simulink model "TDEKF"  (R2020a)
settings: Solver=FixedStepAuto  StartTime=0.0  StopTime=t_sim  FixedStep=0.001  RelTol=1e-3
undefined symbols (not defined in the file or in its folder): initial_acc, initial_position, initial_velocity
libraries: simulink x2
settings Model: Creator=addsd  LastModifiedBy=addsd
settings SFSimCC: CustomCodeUndefinedFunction=UseInterfaceOnly

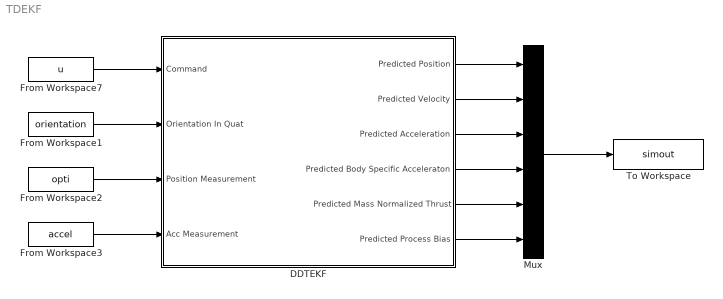
== system TDEKF ==
  DDTEKF : Subsystem  TreatAsAtomicUnit=on  mask{pos_init=initial_position, vel_init=initial_velocity, bsa_init=initial_acc, P_init=eye(11)*0.1, sig_acc=[0.0106 0.0116 0.02554], sig_pos=[0.00001 0.00001 0.00001], sig_quat=[0.001 0.001 0.001 0.001], sig_u=0.001}
      mask prompts: pos_init "Initial Position"; vel_init "Initial Velocity"; bsa_init "Initial Body Specific Acceleration"; P_init "Initial Covariance"; sig_acc "Accelerometer Variance"; sig_pos "Position Sensor Variance"; sig_quat "Orientation Measurement Variance"; sig_u "Process Variance"
      mask help:
      | DDTEKF For Qdrone 1234, dt set to 0.001, gravity vector set to [0 0 9.78909]
      | The Identified Parameters:
      | Kmz = 0.294861
      | Tmz = 0.017707
      | Td = [1.1629 1.1629 0.579374]
      mask init:
      | x_init = [pos_init vel_init bsa_init 5.8033 0]';
      | Q = diag([sig_u sig_quat]);
      | Q_tune = eye(11)*1e-6;
      | Q_tune(1:3, 1:3) = eye(3)*1e-6;
      | Q_tune(4:6, 4:6) = eye(3)*1e-5;
      | Q_tune(7:9, 7:9) = eye(3)*1e-4;
      | % Q_tune(10,10) = 1e-3;
      | Q_tune(11,11) = 1e-4;
      | 
      | dHpos = zeros(3,11);
      | dHpos(1:3, 1:3) = eye(3);
      | Rpos = diag(sig_pos).*eye(3);
      | dHacc = zeros(3,11);
      | dHacc(1:3, 7:9) = eye(3);
      | Racc = diag(sig_acc).*eye(3);
  From Workspace1 : FromWorkspace  VariableName=orientation
  From Workspace2 : FromWorkspace  VariableName=opti
  From Workspace3 : FromWorkspace  VariableName=accel
  From Workspace7 : FromWorkspace  VariableName=u
  Mux : Mux  Inputs=[3 3 3 3 1 1]
  To Workspace : ToWorkspace  VariableName=simout  SaveFormat=Timeseries  SampleTime=-1
  wires:
  DDTEKF/2(Predicted Velocity) -> Mux/2
  DDTEKF/4(Predicted Body Specific Acceleraton) -> Mux/4
  DDTEKF/6(Predicted Process Bias) -> Mux/6
  Mux/1 -> To Workspace/1
  DDTEKF/1(Predicted Position) -> Mux/1
  DDTEKF/3(Predicted Acceleration) -> Mux/3
  From Workspace3/1 -> DDTEKF/4(Acc Measurement)
  From Workspace2/1 -> DDTEKF/3(Position Measurement)
  DDTEKF/5(Predicted Mass Normalized Thrust) -> Mux/5
  From Workspace7/1 -> DDTEKF/1(Command)
  From Workspace1/1 -> DDTEKF/2(Orientation In Quat)

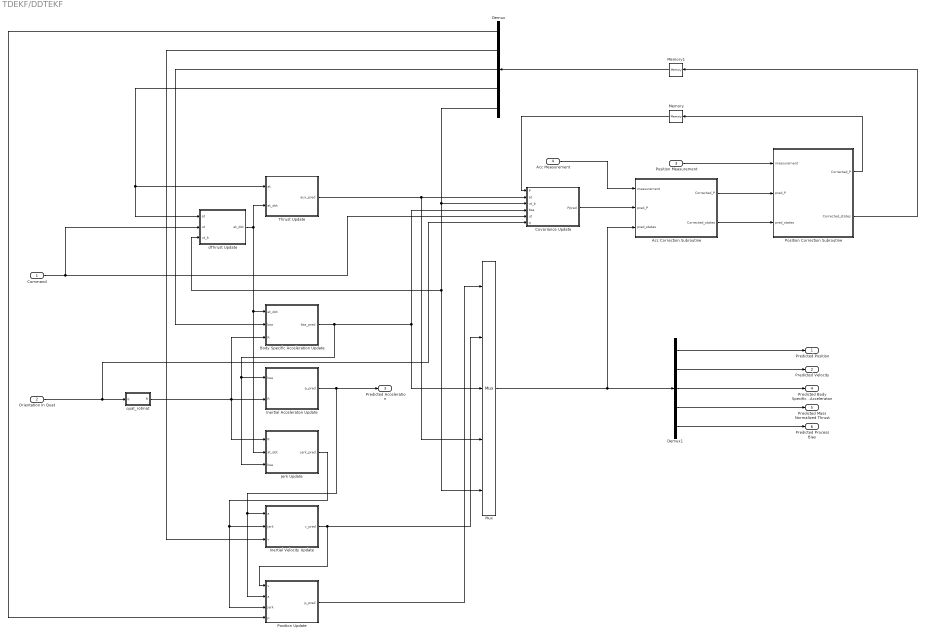
== system TDEKF/DDTEKF ==
  Command : Inport
  Orientation In Quat : Inport  Port=2
  Position Measurement : Inport  Port=3
  Acc Measurement : Inport  Port=4
  Acc Correction Subroutine : Subsystem
  Body Specific Acceleration Update : Subsystem
  Covariance Update : Subsystem
  Demux : Demux  Outputs=[3 3 3 1 1]
  Demux1 : Demux  Outputs=[3 3 3 1 1]
  Inertial Acceleraton Update : Subsystem
  Inertial Velocity Update : Subsystem
  Jerk Update : Subsystem
  Memory : Memory  InitialCondition=P_init
  Memory1 : Memory  InitialCondition=x_init
  Mux : Mux  Inputs=[3 3 3 1 1]
  Position Correction Subroutine : Subsystem  TreatAsAtomicUnit=on  SystemSampleTime=0.001
  Position Update : Subsystem
  Thrust Update : Subsystem
  dThrust Update : Subsystem
  quat_rotmat : Subsystem
  Predicted Position : Outport
  Predicted Velocity : Outport  Port=2
  Predicted Acceleration : Outport  Port=3
  Predicted Body Specific Acceleraton : Outport  Port=4
  Predicted Mass Normalized Thrust : Outport  Port=5
  Predicted Process Bias : Outport  Port=6
  wires:
  dThrust Update/1(at_dot) -> Thrust Update/2(at_dot), Jerk Update/2(at_dot), Body Specific Acceleration Update/1(at_dot)
  Command/1 -> Covariance Update/5(ut), dThrust Update/2(ut)
  Demux/4 -> dThrust Update/1(at), Thrust Update/1(at)
  Demux/5 -> Covariance Update/3(ut_b), dThrust Update/3(ut_b), Mux/5
  Orientation In Quat/1 -> quat_rotmat/1(q), Covariance Update/6(q)
  quat_rotmat/1(R) -> Body Specific Acceleration Update/3(R), Inertial Acceleraton Update/2(R), Jerk Update/1(R)
  Body Specific Acceleration Update/1(bsa_pred) -> Jerk Update/3(bsa), Inertial Acceleraton Update/1(bsa), Covariance Update/4(bsa), Mux/3
  Demux/3 -> Body Specific Acceleration Update/2(bsa)
  Inertial Acceleraton Update/1(a_pred) -> Predicted Acceleration/1, Inertial Velocity Update/1(a), Position Update/2(a)
  Jerk Update/1(jerk_pred) -> Position Update/3(jerk), Inertial Velocity Update/2(jerk)
  Demux/2 -> Inertial Velocity Update/3(v)
  Inertial Velocity Update/1(v_pred) -> Mux/2, Position Update/1(v)
  Demux/1 -> Position Update/4(p)
  Thrust Update/1(aux_pred) -> Mux/4, Covariance Update/2(at)
  Mux/1 -> Demux1/1, Acc Correction Subroutine/3(pred_states)
  Acc Correction Subroutine/1(Corrected_P) -> Position Correction Subroutine/2("pred_P ")
  Acc Correction Subroutine/2(Corrected_states) -> Position Correction Subroutine/3(pred_states)
  Covariance Update/1(Ppred) -> Acc Correction Subroutine/2("pred_P ")
  Memory/1 -> Covariance Update/1(P)
  Memory1/1 -> Demux/1
  Demux1/2 -> Predicted Velocity/1
  Demux1/1 -> Predicted Position/1
  Demux1/3 -> Predicted Body Specific Acceleraton/1
  Demux1/5 -> Predicted Process Bias/1
  Demux1/4 -> Predicted Mass Normalized Thrust/1
  Position Update/1(p_pred) -> Mux/1
  Acc Measurement/1 -> Acc Correction Subroutine/1(measurement)
  Position Measurement/1 -> Position Correction Subroutine/1(measurement)
  Position Correction Subroutine/2(Corrected_states) -> Memory1/1
  Position Correction Subroutine/1(Corrected_P) -> Memory/1

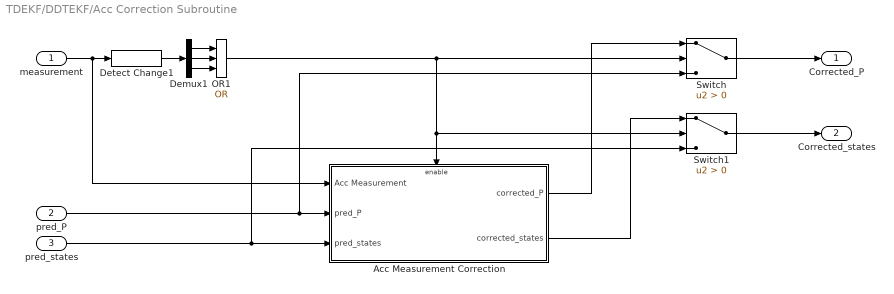
== system TDEKF/DDTEKF/Acc Correction Subroutine ==
  measurement : Inport
  "pred_P " : Inport  Port=2
  pred_states : Inport  Port=3
  Acc Measurement Correction : Subsystem
  Demux1 : Demux  Outputs=3
  Detect Change1 : simulink/Logic and Bit Operations/Detect Change  vinit=[0;0;0]  OutDataTypeStr=boolean
  OR1 : Logic  Operator=OR  Inputs=3  IconShape=distinctive  AllPortsSameDT=off  OutDataTypeStr=boolean
  Switch : Switch  Criteria=u2 > Threshold
  Switch1 : Switch  Criteria=u2 > Threshold
  Corrected_P : Outport
  Corrected_states : Outport  Port=2
  wires:
  Demux1/1 -> OR1/1
  measurement/1 -> Acc Measurement Correction/1(Acc Measurement), Detect Change1/1
  Demux1/3 -> OR1/3
  OR1/1 -> Acc Measurement Correction/Enable, Switch1/2, Switch/2
  Detect Change1/1 -> Demux1/1
  Demux1/2 -> OR1/2
  Switch1/1 -> Corrected_states/1
  "pred_P "/1 -> Switch/3, Acc Measurement Correction/2("pred_P ")
  pred_states/1 -> Switch1/3, Acc Measurement Correction/3(pred_states)
  Acc Measurement Correction/2(corrected_states) -> Switch1/1
  Switch/1 -> Corrected_P/1
  Acc Measurement Correction/1(corrected_P) -> Switch/1

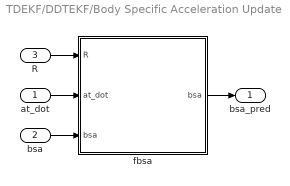
== system TDEKF/DDTEKF/Body Specific Acceleration Update ==
  at_dot : Inport
  bsa : Inport  Port=2
  R : Inport  Port=3
  fbsa : MATLAB Function  TreatAsAtomicUnit=on
  bsa_pred : Outport
  wires:
  fbsa/1(bsa) -> bsa_pred/1
  R/1 -> fbsa/1(R)
  at_dot/1 -> fbsa/2(at_dot)
  bsa/1 -> fbsa/3("bsa ")

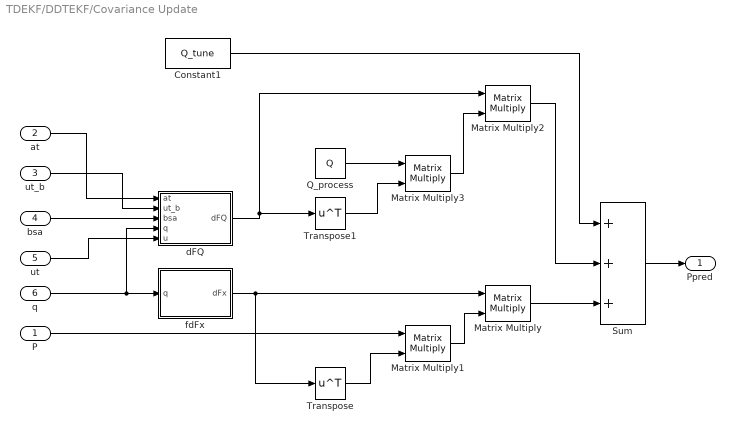
== system TDEKF/DDTEKF/Covariance Update ==
  P : Inport
  at : Inport  Port=2
  ut_b : Inport  Port=3
  bsa : Inport  Port=4
  ut : Inport  Port=5
  q : Inport  Port=6
  Constant1 : Constant  Value=Q_tune
  Matrix Multiply{,1..3} (4 alike) : Product  Multiplication=Matrix(*)
  Q_process : Constant  Value=Q
  Sum : Sum  Inputs=+++
  Transpose : Math  Operator=transpose  SaturateOnIntegerOverflow=on
  Transpose1 : Math  Operator=transpose  SaturateOnIntegerOverflow=on
  dFQ : MATLAB Function  TreatAsAtomicUnit=on
  fdFx : MATLAB Function  TreatAsAtomicUnit=on
  Ppred : Outport
  wires:
  Matrix Multiply3/1 -> Matrix Multiply2/2
  Transpose1/1 -> Matrix Multiply3/2
  Matrix Multiply1/1 -> Matrix Multiply/2
  fdFx/1(dFx) -> Transpose/1, Matrix Multiply/1
  Transpose/1 -> Matrix Multiply1/2
  Q_process/1 -> Matrix Multiply3/1
  dFQ/1(dFQ) -> Matrix Multiply2/1, Transpose1/1
  ut/1 -> dFQ/5(u)
  Matrix Multiply/1 -> Sum/3
  Sum/1 -> Ppred/1
  Constant1/1 -> Sum/1
  q/1 -> dFQ/4(q), fdFx/1(q)
  at/1 -> dFQ/1(at)
  ut_b/1 -> dFQ/2(ut_b)
  bsa/1 -> dFQ/3(bsa)
  P/1 -> Matrix Multiply1/1
  Matrix Multiply2/1 -> Sum/2

== system TDEKF/DDTEKF/Inertial Acceleraton Update ==
  bsa : Inport
  R : Inport  Port=2
  fa : MATLAB Function  TreatAsAtomicUnit=on
  a_pred : Outport
  wires:
  fa/1(fa) -> a_pred/1
  R/1 -> fa/1(R)
  bsa/1 -> fa/2(bsa)

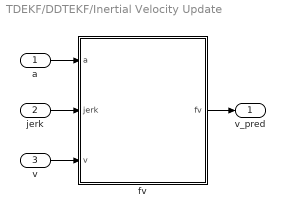
== system TDEKF/DDTEKF/Inertial Velocity Update ==
  a : Inport
  jerk : Inport  Port=2
  v : Inport  Port=3
  fv : MATLAB Function  TreatAsAtomicUnit=on
  v_pred : Outport
  wires:
  fv/1(fv) -> v_pred/1
  a/1 -> fv/1(a)
  jerk/1 -> fv/2(jerk)
  v/1 -> fv/3(v)

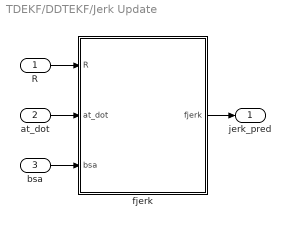
== system TDEKF/DDTEKF/Jerk Update ==
  R : Inport
  at_dot : Inport  Port=2
  bsa : Inport  Port=3
  fjerk : MATLAB Function  TreatAsAtomicUnit=on
  jerk_pred : Outport
  wires:
  fjerk/1(fjerk) -> jerk_pred/1
  bsa/1 -> fjerk/3(bsa)
  at_dot/1 -> fjerk/2(at_dot)
  R/1 -> fjerk/1(R)

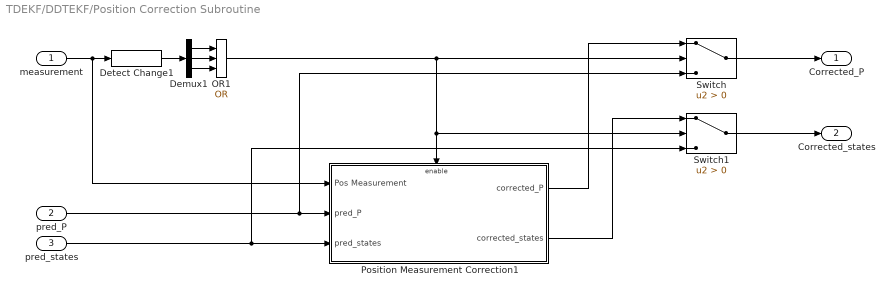
== system TDEKF/DDTEKF/Position Correction Subroutine ==
  measurement : Inport
  "pred_P " : Inport  Port=2
  pred_states : Inport  Port=3
  Demux1 : Demux  Outputs=3
  Detect Change1 : simulink/Logic and Bit Operations/Detect Change  vinit=[0;0;0]  OutDataTypeStr=boolean
  OR1 : Logic  Operator=OR  Inputs=3  IconShape=distinctive  AllPortsSameDT=off  OutDataTypeStr=boolean
  Position Measurement Correction1 : Subsystem
  Switch : Switch  Criteria=u2 > Threshold
  Switch1 : Switch  Criteria=u2 > Threshold
  Corrected_P : Outport
  Corrected_states : Outport  Port=2
  wires:
  Demux1/1 -> OR1/1
  measurement/1 -> Position Measurement Correction1/1(Pos Measurement), Detect Change1/1
  Demux1/3 -> OR1/3
  Detect Change1/1 -> Demux1/1
  Demux1/2 -> OR1/2
  Switch1/1 -> Corrected_states/1
  "pred_P "/1 -> Position Measurement Correction1/2("pred_P "), Switch/3
  pred_states/1 -> Position Measurement Correction1/3(pred_states), Switch1/3
  Position Measurement Correction1/2(corrected_states) -> Switch1/1
  Switch/1 -> Corrected_P/1
  Position Measurement Correction1/1(corrected_P) -> Switch/1
  OR1/1 -> Position Measurement Correction1/Enable, Switch1/2, Switch/2

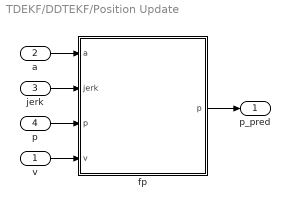
== system TDEKF/DDTEKF/Position Update ==
  v : Inport
  a : Inport  Port=2
  jerk : Inport  Port=3
  p : Inport  Port=4
  fp : MATLAB Function  TreatAsAtomicUnit=on
  p_pred : Outport
  wires:
  fp/1(p) -> p_pred/1
  a/1 -> fp/1(a)
  jerk/1 -> fp/2(jerk)
  v/1 -> fp/4(v)
  p/1 -> fp/3("p ")

== system TDEKF/DDTEKF/Thrust Update ==
  at : Inport
  at_dot : Inport  Port=2
  Gain : Gain  Gain=1/1.0e+3
  Sum : Sum  Inputs=|++
  aux_pred : Outport
  wires:
  at_dot/1 -> Gain/1
  Gain/1 -> Sum/2
  at/1 -> Sum/1
  Sum/1 -> aux_pred/1

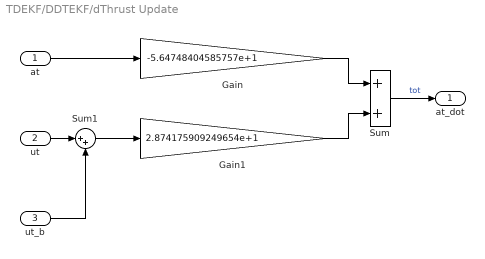
== system TDEKF/DDTEKF/dThrust Update ==
  at : Inport
  ut : Inport  Port=2
  ut_b : Inport  Port=3
  Gain : Gain  Gain=-5.64748404585757e+1
  Gain1 : Gain  Gain=2.874175909249654e+1
  Sum : Sum
  Sum1 : Sum  Inputs=|++
  at_dot : Outport
  wires:
  Sum/1 -> at_dot/1  "tot"
  at/1 -> Gain/1
  Gain/1 -> Sum/1
  Gain1/1 -> Sum/2
  Sum1/1 -> Gain1/1
  ut/1 -> Sum1/1
  ut_b/1 -> Sum1/2

== system TDEKF/DDTEKF/quat_rotmat ==
  q : Inport
  Signal Specification : SignalSpecification  Dimensions=[3 3]
  quat_rotmat : MATLAB Function  TreatAsAtomicUnit=on
  R : Outport
  wires:
  quat_rotmat/1(y) -> Signal Specification/1
  Signal Specification/1 -> R/1
  q/1 -> quat_rotmat/1(u)

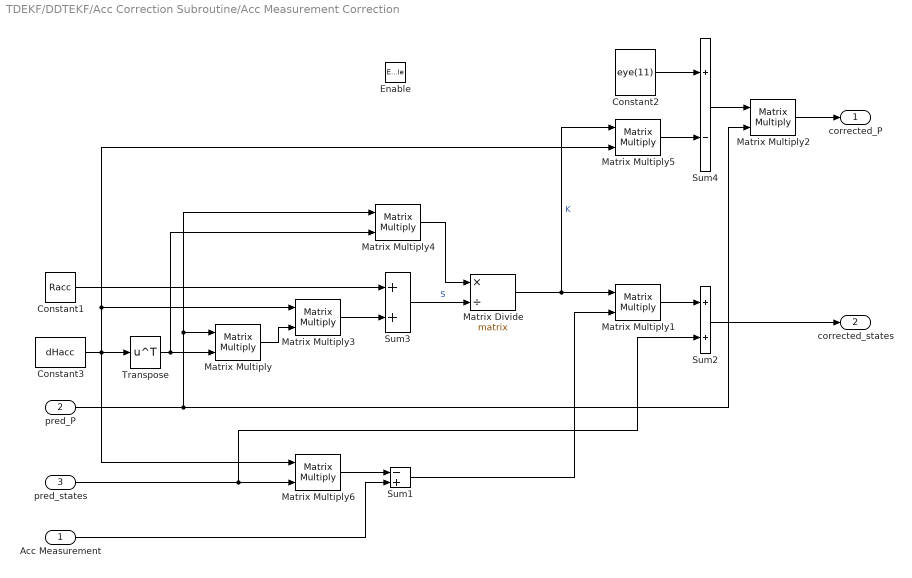
== system TDEKF/DDTEKF/Acc Correction Subroutine/Acc Measurement Correction ==
  Acc Measurement : Inport
  "pred_P " : Inport  Port=2
  pred_states : Inport  Port=3
  Enable : EnablePort
  Constant1 : Constant  Value=Racc
  Constant2 : Constant  Value=eye(11)
  Constant3 : Constant  Value=dHacc
  Matrix Divide : Product  Inputs=*/  Multiplication=Matrix(*)
  Matrix Multiply{,1..6} (7 alike) : Product  Multiplication=Matrix(*)
  Sum1 : Sum  Inputs=-+
  Sum2 : Sum
  Sum3 : Sum
  Sum4 : Sum  Inputs=+-
  Transpose : Math  Operator=transpose  SaturateOnIntegerOverflow=on
  corrected_P : Outport
  corrected_states : Outport  Port=2
  wires:
  Constant3/1 -> Matrix Multiply6/1, Matrix Multiply5/2, Matrix Multiply3/1, Transpose/1
  Matrix Multiply4/1 -> Matrix Divide/1
  Sum3/1 -> Matrix Divide/2  "S"
  Matrix Multiply/1 -> Matrix Multiply3/2
  Matrix Multiply3/1 -> Sum3/2
  Transpose/1 -> Matrix Multiply4/2, Matrix Multiply/2
  Constant1/1 -> Sum3/1
  Matrix Multiply6/1 -> Sum1/1
  Acc Measurement/1 -> Sum1/2
  pred_states/1 -> Sum2/2, Matrix Multiply6/2
  Matrix Divide/1 -> Matrix Multiply5/1, Matrix Multiply1/1  "K"
  Sum1/1 -> Matrix Multiply1/2
  Matrix Multiply1/1 -> Sum2/1
  Sum2/1 -> corrected_states/1
  Matrix Multiply5/1 -> Sum4/2
  Sum4/1 -> Matrix Multiply2/1
  Constant2/1 -> Sum4/1
  Matrix Multiply2/1 -> corrected_P/1
  "pred_P "/1 -> Matrix Multiply2/2, Matrix Multiply4/1, Matrix Multiply/1

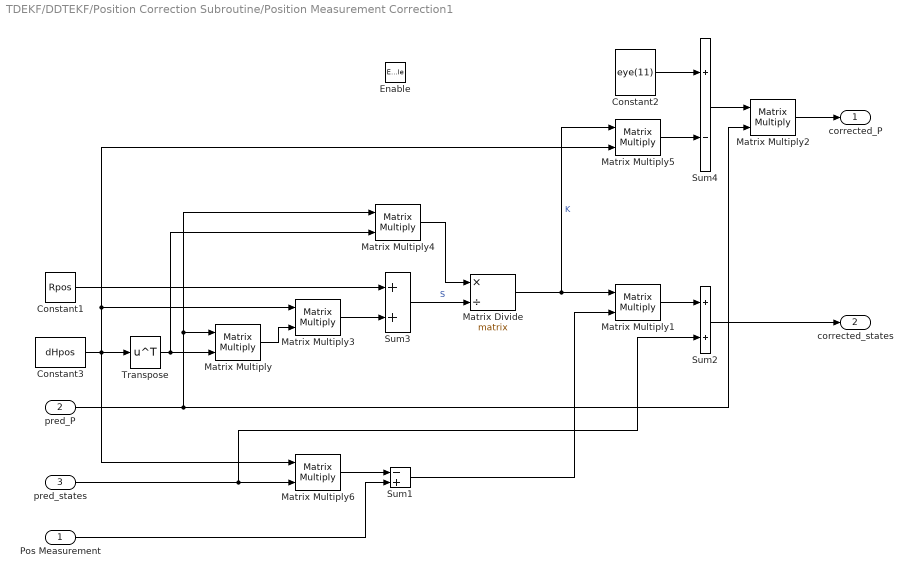
== system TDEKF/DDTEKF/Position Correction Subroutine/Position Measurement Correction1 ==
  Pos Measurement : Inport
  "pred_P " : Inport  Port=2
  pred_states : Inport  Port=3
  Enable : EnablePort
  Constant1 : Constant  Value=Rpos
  Constant2 : Constant  Value=eye(11)
  Constant3 : Constant  Value=dHpos
  Matrix Divide : Product  Inputs=*/  Multiplication=Matrix(*)
  Matrix Multiply{,1..6} (7 alike) : Product  Multiplication=Matrix(*)
  Sum1 : Sum  Inputs=-+
  Sum2 : Sum
  Sum3 : Sum
  Sum4 : Sum  Inputs=+-
  Transpose : Math  Operator=transpose  SaturateOnIntegerOverflow=on
  corrected_P : Outport
  corrected_states : Outport  Port=2
  wires:
  Sum3/1 -> Matrix Divide/2  "S"
  Matrix Multiply1/1 -> Sum2/1
  "pred_P "/1 -> Matrix Multiply2/2, Matrix Multiply4/1, Matrix Multiply/1
  pred_states/1 -> Sum2/2, Matrix Multiply6/2
  Matrix Multiply5/1 -> Sum4/2
  Transpose/1 -> Matrix Multiply4/2, Matrix Multiply/2
  Sum4/1 -> Matrix Multiply2/1
  Matrix Multiply6/1 -> Sum1/1
  Matrix Multiply2/1 -> corrected_P/1
  Matrix Multiply3/1 -> Sum3/2
  Sum2/1 -> corrected_states/1
  Matrix Divide/1 -> Matrix Multiply5/1, Matrix Multiply1/1  "K"
  Pos Measurement/1 -> Sum1/2
  Constant3/1 -> Matrix Multiply6/1, Matrix Multiply5/2, Matrix Multiply3/1, Transpose/1
  Constant2/1 -> Sum4/1
  Matrix Multiply/1 -> Matrix Multiply3/2
  Matrix Multiply4/1 -> Matrix Divide/1
  Sum1/1 -> Matrix Multiply1/2
  Constant1/1 -> Sum3/1

== matlab function TDEKF/DDTEKF/quat_rotmat/quat_rotmat ==
  data: u input; y output
function y = fcn(u)

if(iscolumn(u))
    t = u';
else
    t = u;
end

y = quat2rotm(t);

end

== matlab function TDEKF/DDTEKF/Covariance Update/dFQ ==
  data: at input; ut_b input; bsa input; q input; u input; dFQ output
function dFQ = fdFQv2(at,ut_b,bsa,q,u)
%FDFQV2
%    DFQ = FDFQV2(R(3,1),R(3,2),R(3,3),AUX,AUX_B,bsa(1),bsa(2),bsa(3),q(1),q(2),q(3),q(4),U)

%    This function was generated by the Symbolic Math Toolbox version 8.5.
%    23-May-2021 09:26:08

R = quat2rotm(q');
t2 = q(1).^2;
t3 = q(2).^2;
t4 = q(3).^2;
t5 = q(4).^2;
t6 = -bsa(1);
t7 = -bsa(2);
t8 = (bsa(1).*q(1))./5.0e+2;
t9 = (bsa(1).*q(2))./5.0e+2;
t10 = (bsa(2).*q(1))./5.0e+2;
t11 = (bsa(1).*q(3))./5.0e+2;
t12 = (bsa(2).*q(2))./5.0e+2;
t13 = (bsa(3).*q(1))./5.0e+2;
t14 = (bsa(1).*q(4))./5.0e+2;
t15 = (bsa(2).*q(3))./5.0e+2;
t16 = (bsa(3).*q(2))./5.0e+2;
t17 = (bsa(2).*q(4))./5.0e+2;
t18 = (bsa(3).*q(3))./5.0e+2;
t19 = (bsa(3).*q(4))./5.0e+2;
t23 = (bsa(1).*q(1))./1.0e+6;
t24 = (bsa(1).*q(2))./1.0e+6;
t25 = (bsa(2).*q(1))./1.0e+6;
t26 = (bsa(1).*q(3))./1.0e+6;
t27 = (bsa(2).*q(2))./1.0e+6;
t28 = (bsa(3).*q(1))./1.0e+6;
t29 = (bsa(1).*q(4))./1.0e+6;
t30 = (bsa(2).*q(3))./1.0e+6;
t31 = (bsa(3).*q(2))./1.0e+6;
t32 = (bsa(2).*q(4))./1.0e+6;
t33 = (bsa(3).*q(3))./1.0e+6;
t34 = (bsa(3).*q(4))./1.0e+6;
t38 = R(3,1).*9.78909;
t39 = R(3,2).*9.78909;
t40 = bsa(3).*1.726000821576391;
t41 = at.*5.64748404585757e+1;
t42 = R(3,3).*1.689597738248524e+1;
t44 = q(1).*1.683565224868862e-2;
t45 = q(2).*1.683565224868862e-2;
t46 = q(3).*1.683565224868862e-2;
t47 = q(4).*1.683565224868862e-2;
t70 = ut_b.*2.874175909249654e+1;
t71 = u.*2.874175909249654e+1;
t20 = -t11;
t21 = -t16;
t22 = -t17;
t35 = -t26;
t36 = -t31;
t37 = -t32;
t43 = -t42;
t48 = t6+t38;
t49 = t7+t39;
t72 = -t71;
t50 = (q(1).*t48)./1.1629e+6;
t51 = (q(2).*t48)./1.1629e+6;
t52 = (q(1).*t49)./1.1629e+6;
t53 = (q(3).*t48)./1.1629e+6;
t54 = (q(2).*t49)./1.1629e+6;
t55 = (q(4).*t48)./1.1629e+6;
t56 = (q(3).*t49)./1.1629e+6;
t57 = (q(4).*t49)./1.1629e+6;
t60 = (q(1).*t48)./3.4887e+9;
t61 = (q(2).*t48)./3.4887e+9;
t62 = (q(1).*t49)./3.4887e+9;
t63 = (q(3).*t48)./3.4887e+9;
t64 = (q(2).*t49)./3.4887e+9;
t65 = (q(4).*t48)./3.4887e+9;
t66 = (q(3).*t49)./3.4887e+9;
t67 = (q(4).*t49)./3.4887e+9;
t73 = t40+t41+t43+t70+t72;
t58 = -t53;
t59 = -t57;
t68 = -t63;
t69 = -t67;
t74 = (q(1).*t73)./1.0e+6;
t75 = (q(2).*t73)./1.0e+6;
t76 = (q(3).*t73)./1.0e+6;
t77 = (q(4).*t73)./1.0e+6;
t81 = (q(1).*t73)./3.0e+9;
t82 = (q(2).*t73)./3.0e+9;
t83 = (q(3).*t73)./3.0e+9;
t84 = (q(4).*t73)./3.0e+9;
t78 = -t74;
t79 = -t76;
t80 = -t77;
t85 = -t81;
t86 = -t83;
t87 = -t84;
t88 = t10+t14+t21+t52+t55+t75;
t92 = t25+t29+t36+t62+t65+t82;
t89 = t9+t15+t19+t51+t56+t80;
t90 = t12+t13+t20+t54+t58+t78;
t91 = t8+t18+t22+t50+t59+t79;
t93 = t24+t30+t34+t61+t66+t87;
t94 = t27+t28+t35+t64+t68+t85;
t95 = t23+t33+t37+t60+t69+t86;
dFQ = reshape([q(1).*q(3).*9.580586364165514e-9+q(2).*q(4).*9.580586364165514e-9,q(1).*q(2).*(-9.580586364165514e-9)+q(3).*q(4).*9.580586364165514e-9,t2.*4.790293182082757e-9-t3.*4.790293182082757e-9-t4.*4.790293182082757e-9+t5.*4.790293182082757e-9,q(1).*q(3).*2.874175909249654e-5+q(2).*q(4).*2.874175909249654e-5,q(1).*q(2).*(-2.874175909249654e-5)+q(3).*q(4).*2.874175909249654e-5,t2.*1.437087954624827e-5-t3.*1.437087954624827e-5-t4.*1.437087954624827e-5+t5.*1.437087954624827e-5,0.0,0.0,2.874175909249654e-2,2.874175909249654e-2,0.0,t95,t92,t94,t91,t88,t90,-t46,t45,q(1).*3.379195476497047e-2,0.0,0.0,t93,t26-t27-t28+t63-t64+t81,t92,t89,t11-t12-t13+t53-t54+t74,t88,t47,t44,q(2).*(-3.379195476497047e-2),0.0,0.0,t94,t93,-t23+t32-t33-t60+t67+t83,t90,t89,-t8+t17-t18-t50+t57+t76,-t44,t47,q(3).*(-3.379195476497047e-2),0.0,0.0,-t25-t29+t31-t62-t65-t82,t95,t93,-t10-t14+t16-t52-t55-t75,t91,t89,t45,t46,q(4).*3.379195476497047e-2,0.0,0.0],[11,5]);

== matlab function TDEKF/DDTEKF/Covariance Update/fdFx ==
  data: q input; dFx output
function dFx = fdFxv2(q)
%FDFXV2
%    DFX = FDFXV2(Q1,Q2,Q3,Q4)

%    This function was generated by the Symbolic Math Toolbox version 8.5.
%    23-May-2021 09:26:06

t2 = q(1).^2;
t3 = q(2).^2;
t4 = q(3).^2;
t5 = q(4).^2;
t6 = q(1).*q(4).*1.999140080832402e-3;
t7 = q(2).*q(3).*1.999140080832402e-3;
t13 = q(1).*q(4).*9.997133602774673e-7;
t14 = q(2).*q(3).*9.997133602774673e-7;
t8 = t2.*9.995700404162009e-4;
t9 = t3.*9.995700404162009e-4;
t10 = t4.*9.995700404162009e-4;
t11 = t5.*9.995700404162009e-4;
t15 = t2.*4.998566801387336e-7;
t16 = t3.*4.998566801387336e-7;
t17 = t4.*4.998566801387336e-7;
t18 = t5.*4.998566801387336e-7;
t12 = -t11;
t19 = -t18;
dFx = reshape([1.0,0.0,0.0,0.0,0.0,0.0,0.0,0.0,0.0,0.0,0.0,0.0,1.0,0.0,0.0,0.0,0.0,0.0,0.0,0.0,0.0,0.0,0.0,0.0,1.0,0.0,0.0,0.0,0.0,0.0,0.0,0.0,0.0,1.0./1.0e+3,0.0,0.0,1.0,0.0,0.0,0.0,0.0,0.0,0.0,0.0,0.0,1.0./1.0e+3,0.0,0.0,1.0,0.0,0.0,0.0,0.0,0.0,0.0,0.0,0.0,1.0./1.0e+3,0.0,0.0,1.0,0.0,0.0,0.0,0.0,0.0,t15+t16-t17+t19,t13+t14,q(1).*q(3).*(-9.997133602774673e-7)+q(2).*q(4).*9.997133602774673e-7,t8+t9-t10+t12,t6+t7,q(1).*q(3).*(-1.999140080832402e-3)+q(2).*q(4).*1.999140080832402e-3,9.991400808324018e-1,0.0,0.0,0.0,0.0,-t13+t14,t15-t16+t17+t19,q(1).*q(2).*9.997133602774673e-7+q(3).*q(4).*9.997133602774673e-7,-t6+t7,t8-t9+t10+t12,q(1).*q(2).*1.999140080832402e-3+q(3).*q(4).*1.999140080832402e-3,0.0,9.991400808324018e-1,0.0,0.0,0.0,q(1).*q(3).*9.994246663928079e-7+q(2).*q(4).*9.994246663928079e-7,q(1).*q(2).*(-9.994246663928079e-7)+q(3).*q(4).*9.994246663928079e-7,t2.*4.997123331964039e-7-t3.*4.997123331964039e-7-t4.*4.997123331964039e-7+t5.*4.997123331964039e-7,q(1).*q(3).*1.998273999178424e-3+q(2).*q(4).*1.998273999178424e-3,q(1).*q(2).*(-1.998273999178424e-3)+q(3).*q(4).*1.998273999178424e-3,t2.*9.991369995892118e-4-t3.*9.991369995892118e-4-t4.*9.991369995892118e-4+t5.*9.991369995892118e-4,0.0,0.0,9.982739991784236e-1,0.0,0.0,q(1).*q(3).*(-1.882494681952523e-8)-q(2).*q(4).*1.882494681952523e-8,q(1).*q(2).*1.882494681952523e-8-q(3).*q(4).*1.882494681952523e-8,t2.*(-9.412473409762617e-9)+t3.*9.412473409762617e-9+t4.*9.412473409762617e-9-t5.*9.412473409762617e-9,q(1).*q(3).*(-5.64748404585757e-5)-q(2).*q(4).*5.64748404585757e-5,q(1).*q(2).*5.64748404585757e-5-q(3).*q(4).*5.64748404585757e-5,t2.*(-2.823742022928785e-5)+t3.*2.823742022928785e-5+t4.*2.823742022928785e-5-t5.*2.823742022928785e-5,0.0,0.0,-5.64748404585757e-2,9.435251595414243e-1,0.0,q(1).*q(3).*(-9.580586364165514e-9)-q(2).*q(4).*9.580586364165514e-9,q(1).*q(2).*9.580586364165514e-9-q(3).*q(4).*9.580586364165514e-9,t2.*(-4.790293182082757e-9)+t3.*4.790293182082757e-9+t4.*4.790293182082757e-9-t5.*4.790293182082757e-9,q(1).*q(3).*(-2.874175909249654e-5)-q(2).*q(4).*2.874175909249654e-5,q(1).*q(2).*2.874175909249654e-5-q(3).*q(4).*2.874175909249654e-5,t2.*(-1.437087954624827e-5)+t3.*1.437087954624827e-5+t4.*1.437087954624827e-5-t5.*1.437087954624827e-5,0.0,0.0,-2.874175909249654e-2,-2.874175909249654e-2,1.0],[11,11]);

== matlab function TDEKF/DDTEKF/Body Specific Acceleration Update/fbsa ==
  data: R input; bsa output; at_dot input; bsa input
function bsa = fbsa(R, at_dot, bsa)
%FBSA
%    FBSA = FBSA(R(3, 1),R(3, 2),R(3, 3),AUX_DOT,BSA1,BSA2,BSA3)

%    This function was generated by the Symbolic Math Toolbox version 8.5.
%    01-Apr-2021 15:55:23

bsa = [R(3, 1).*8.417826124344312e-3+bsa(1).*9.991400808324018e-1;R(3, 2).*8.417826124344312e-3+bsa(2).*9.991400808324018e-1;R(3, 3).*1.689597738248524e-2+at_dot./1.0e+3+bsa(3).*9.982739991784236e-1];

== matlab function TDEKF/DDTEKF/Inertial Acceleraton Update/fa ==
  data: R input; fa output; bsa input
function fa = fa(R,bsa)
%FAV2
%    FA = FAV2(R(1,1),R(1,2),R(1,3),R(2,1),R(2,2),R(2,3),R(3,1),R(3,2),R(3,3),bsa(1),bsa(2),bsa(3))

%    This function was generated by the Symbolic Math Toolbox version 8.5.
%    23-May-2021 09:26:09

fa = [R(1,1).*bsa(1)+R(1,2).*bsa(2)+R(1,3).*bsa(3);R(2,1).*bsa(1)+R(2,2).*bsa(2)+R(2,3).*bsa(3);R(3,1).*bsa(1)+R(3,2).*bsa(2)+R(3,3).*bsa(3)-9.78909];

== matlab function TDEKF/DDTEKF/Inertial Velocity Update/fv ==
  data: a input; fv output; jerk input; v input
function fv = fv(a, jerk, v)
%FV
%    FV = FV(A1,A2,A3,JERK1,JERK2,JERK3,V1,V2,V3)

%    This function was generated by the Symbolic Math Toolbox version 8.5.
%    01-Apr-2021 16:03:03

fv = [a(1)./1.0e+3+jerk(1)./2.0e+6+v(1);a(2)./1.0e+3+jerk(2)./2.0e+6+v(2);a(3)./1.0e+3+jerk(3)./2.0e+6+v(3)];

== matlab function TDEKF/DDTEKF/Position Update/fp ==
  data: a input; p output; jerk input; p input; v input
function p = fcn(a, jerk, p, v)
%FP
%    FP = FP(A1,A2,A3,JERK1,JERK2,JERK3,P1,P2,P3,V1,V2,V3)

%    This function was generated by the Symbolic Math Toolbox version 8.5.
%    01-Apr-2021 16:05:23

p = [a(1)./2.0e+6+jerk(1)./6.0e+9+p(1)+v(1)./1.0e+3;a(2)./2.0e+6+jerk(2)./6.0e+9+p(2)+v(2)./1.0e+3;a(3)./2.0e+6+jerk(3)./6.0e+9+p(3)+v(3)./1.0e+3];

== matlab function TDEKF/DDTEKF/Jerk Update/fjerk ==
  data: R input; at_dot input; fjerk output; bsa input
function fjerk = fjerk(R,at_dot,bsa)
%FJERKV2
%    FJERK = FJERKV2(R(1,1),R(1,2),R(1,3),R(2,1),R(2,2),R(2,3),R(3,1),R(3,2),R(3,3),at_dot,bsa(1),bsa(2),bsa(3))

%    This function was generated by the Symbolic Math Toolbox version 8.5.
%    23-May-2021 09:26:09

t2 = -bsa(1);
t3 = -bsa(2);
t4 = R(3,1).*9.78909;
t5 = R(3,2).*9.78909;
t6 = bsa(3).*1.726000821576391;
t8 = R(3,3).*1.689597738248524e+1;
t7 = -t6;
t9 = t2+t4;
t10 = t3+t5;
t11 = at_dot+t7+t8;
fjerk = [R(1,1).*t9.*8.599191675982458e-1+R(1,2).*t10.*8.599191675982458e-1+R(1,3).*t11;R(2,1).*t9.*8.599191675982458e-1+R(2,2).*t10.*8.599191675982458e-1+R(2,3).*t11;R(3,1).*t9.*8.599191675982458e-1+R(3,2).*t10.*8.599191675982458e-1+R(3,3).*t11];
